simulink model "SUB_IC_Fcn_Welcome"  (R2018b)
settings: Solver=VariableStepDiscrete  StartTime=0.0  StopTime=10  RelTol=1e-3
PreLoadFcn:
  | if(exist('MBDS_ModelCallback', 'file'))
  |    MBDS_ModelCallback('PreLoad');
  | end
PostLoadFcn:
  | if(exist('MBDS_ModelCallback', 'file'))
  |    MBDS_ModelCallback('PostLoad');
  | end
InitFcn:
  | if(exist('MBDS_ModelCallback', 'file'))
  |    MBDS_ModelCallback('Init');
  | end
StartFcn:
  | if(exist('MBDS_ModelCallback', 'file'))
  |    MBDS_ModelCallback('Start');
  | end
StopFcn:
  | if(exist('MBDS_ModelCallback', 'file'))
  |    MBDS_ModelCallback('Stop');
  | end
undefined symbols (not defined in the file): nbo_False, nbo_True, sigbuilder_block
libraries: simulink x1
PreSaveFcn:
  | if(exist('MBDS_ModelCallback', 'file'))
  |    MBDS_ModelCallback('PreSave');
  | end
CloseFcn:
  | if(exist('MBDS_ModelCallback', 'file'))
  |    MBDS_ModelCallback('Close');
  | end
Description:
  | Design model of an MBDS Subsystem
settings Model: IsTargetCode=false  MBDS_Version=08.20  PauseTimes=0.1  Creator=Marcio Kopke (uid96494)  LastModifiedBy=uie79669
settings ConfigSet: Description=MBDS configuration set optimized for simulation of model designs for automotive embedded systems.
settings SolverCC: MinimalZcImpactIntegration=on
settings DataIOCC: MaxDataPoints=100  SaveFormat=StructureWithTime  SaveOutput=off  DSMLogging=off  VisualizeSimOutput=off  SaveTime=off  SignalLoggingName=LogSignals
settings OptimizationCC: UseDivisionForNetSlopeComputation=UseDivisionForReciprocalsOfIntegersOnly  UseFloatMulNetSlope=on  DefaultUnderspecifiedDataType=single  OptimizeBlockIOStorage=off  BufferReuse=off  GlobalBufferReuse=off  StrengthReduction=on  ExpressionFolding=off  ExpressionDepthLimit=2147483647  LocalBlockOutputs=off  EfficientFloat2IntCast=on  LifeSpan=inf  BufferReusableBoundary=off  OptimizeBlockOrder=speed  OptimizeDataStoreBuffers=off  BusAssignmentInplaceUpdate=off  LabelGuidedReuse=on
settings DebuggingCC: SignalInfNanChecking=error  AlgebraicLoopMsg=error  ArtificialAlgebraicLoopMsg=error  UnderspecifiedInitializationDetection=Classic  CheckExecutionContextPreStartOutputMsg=on  CheckExecutionContextRuntimeOutputMsg=on  BlockPriorityViolationMsg=error  MinStepSizeMsg=error  TimeAdjustmentMsg=warning  SolverPrmCheckMsg=error  InheritedTsInSrcMsg=none  SingleTaskRateTransMsg=error  TasksWithSamePriorityMsg=error  SigSpecEnsureSampleTimeMsg=error  CheckMatrixSingularityMsg=error  ParameterUnderflowMsg=error  ParameterTunabilityLossMsg=error  FixptConstUnderflowMsg=warning  FixptConstOverflowMsg=warning  FixptConstPrecisionLossMsg=warning  VectorMatrixConversionMsg=error  SignalLabelMismatchMsg=warning  SFcnCompatibilityMsg=error  FrameProcessingCompatibilityMsg=warning  UniqueDataStoreMsg=error  BusObjectLabelMismatch=error  RootOutportRequireBusObject=error  AllowSymbolicDim=off  ModelReferenceIOMsg=error  ModelReferenceIOMismatchMessage=error  UnknownTsInhSupMsg=error  ModelReferenceDataLoggingMessage=error  StateNameClashWarn=warning  SimStateOlderReleaseMsg=warning  StrictBusMsg=ErrorOnBusTreatedAsVector  NonBusSignalsTreatedAsBus=error  SFInvalidInputDataAccessInChartInitDiag=error  SFTransitionOutsideNaturalParentDiag=error  SFUnreachableExecutionPathDiag=error  SFUndirectedBroadcastEventsDiag=error  SFTransitionActionBeforeConditionDiag=error  SFTemporalDelaySmallerThanSampleTimeDiag=error  SFExecutionAtInitializationDiag=none
settings HardwareCC: ProdBitPerPointer=32  ProdBitPerSizeT=32  ProdBitPerPtrDiffT=32  ProdLargestAtomicInteger=Long  ProdEndianess=BigEndian  ProdWordSize=32  ProdLongLongMode=on  ProdHWDeviceType=Custom Processor  TargetHWDeviceType=32-bit Generic
settings ModelReferenceCC: PropagateSignalLabelsOutOfModel=off
settings SFSimCC: SimUseLocalCustomCode=off  SimGenImportedTypeDefs=on  CompileTimeRecursionLimit=0  EnableRuntimeRecursion=off  MATLABDynamicMemAlloc=off  DefaultCustomCodeFunctionArrayLayout=Column-major
settings RTWCC: SystemTargetFile=MBDS.tlc  GenCodeOnly=on  TemplateMakefile=MBDS.tmf  Description=MBDS Target  GenerateReport=on  RTWUseLocalCustomCode=off  IncludeHyperlinkInReport=on  LaunchReport=on  GenerateTraceReport=on  GenerateTraceReportSl=on  GenerateTraceReportSf=on  GenerateTraceReportEml=on  GenerateCodeMetricsReport=on  RTWCompilerOptimization=on
settings CodeAppCC: ForceParamTrailComments=on  IgnoreCustomStorageClasses=off  OperatorAnnotations=on  SimulinkDataObjDesc=on  SFDataObjDesc=on  MangleLength=2  CustomSymbolStrType=$N$R$M  CustomSymbolStrFcn=$R$M  CustomSymbolStrUtil=$n$C  InsertBlockDesc=on  StateflowObjectComments=on  MATLABSourceComments=on  ReqsInCode=on  UseSimReservedNames=on
settings STFCustomTargetCC: UtilityFuncGeneration=Shared location  MultiwordLength=256  DynamicStringBufferSize=2  InferredTypesCompatibility=on  ModelReferenceCompliant=off  IncludeMdlTerminateFcn=off  CombineOutputUpdateFcns=on  CombineSignalStateStructs=on  SuppressErrorStatus=on  ERTCustomFileBanners=on  SupportComplex=off  SupportContinuousTime=off  SupportNonInlinedSFcns=off  RemoveDisableFunc=on  RemoveResetFunc=on  ParenthesesLevel=Maximum  CastingMode=Standards  MATLABClassNameForMDSCustomization=Simulink.SoftwareTarget.ERTCustomization  GenerateSharedConstants=off  SystemTargetFile=MBDS.tlc
settings ERTTargetCC: UtilityFuncGeneration=Shared location  DynamicStringBufferSize=2  InferredTypesCompatibility=on  ModelReferenceCompliant=off  ParMdlRefBuildCompliant=off  CompOptLevelCompliant=off  ConcurrentExecutionCompliant=off  IncludeMdlTerminateFcn=off  CombineSignalStateStructs=on  SuppressErrorStatus=on  SupportComplex=off  RemoveDisableFunc=on  ParenthesesLevel=Maximum  CastingMode=Standards  ModelStepFunctionPrototypeControlCompliant=off  CPPClassGenCompliant=off  UseToolchainInfoCompliant=off  GenerateSharedConstants=off  ERTCustomFileTemplate=example_file_process.tlc  EnableDataOwnership=on  PreserveExpressionOrder=on  PreserveIfCondition=on  SuppressUnreachableDefaultCases=off  EnableSignedLeftShifts=off  EnableSignedRightShifts=off  IndentStyle=Allman  NewlineStyle=CR+LF
settings ConfigComp: CovScope=ReferencedModels  CovIncludeTopModel=off  CovPath=SUB_IC_Fcn_Welcome/Model/SUB_IC_Fcn_Welcome_  CovSaveName=covData  CovMetricSettings=dsw  CovFilter=MBDS_CoverageFilter  CovHTMLOptions=-sRT=1 -sVT=0 -aTS=1 -bRG=1 -bTC=1 -hTR=1 -nFC=0 -nFD=0 -scm=1 -bcm=1 -xEv=0 -xEM=1  CovHtmlReporting=on  CovSaveOutputData=off  CovDataFileName=covData  CovShowResultsExplorer=off  CovExternalEMLEnable=off  CovSFcnEnable=off

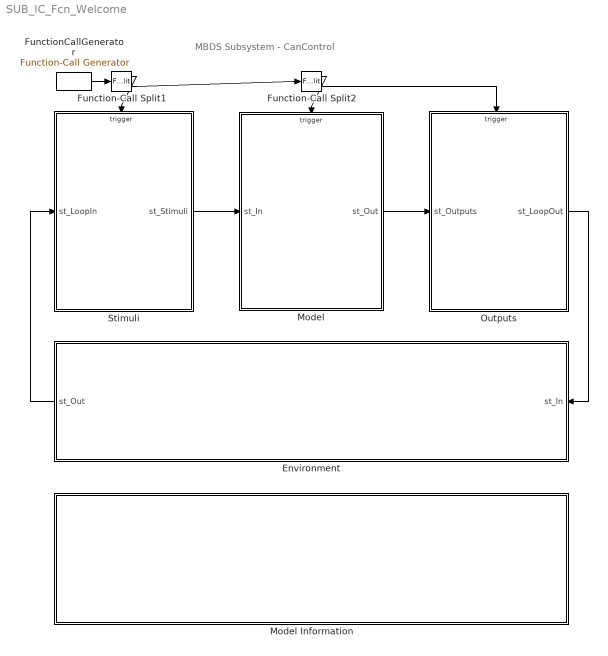
== system SUB_IC_Fcn_Welcome ==
  note: MBDS Subsystem - CanControl
  Environment : Subsystem  Description=Environment subsystem for a MBDS model.
  Function-Call Split1 : FunctionCallSplit  InitFcn=|  NumOutputPorts=2
      | try
      |    MBDS_BlockCallback('Update', gcb);
      | end
      | try
      |    MBDS_BlockCallback('Update', gcb);
      | end
  Function-Call Split2 : FunctionCallSplit  InitFcn=|  NumOutputPorts=2
      | try
      |    MBDS_BlockCallback('Update', gcb);
      | end
      | try
      |    MBDS_BlockCallback('Update', gcb);
      | end
  FunctionCallGenerator : simulink/Ports & Subsystems/Function-Call Generator  sample_time=0.01  numberOfIterations=1
      settings: AttributesFormatString=Ts = %<sample_time>
  Model : Subsystem  Description=Model subsystem for a MBDS model. Here, the input signals to the model functionality are resolved from the Stimuli bus and the output signals of the model functionality are summarized into the Results bus.
  Model Information : Subsystem  InitFcn=|  mask(ModelInformation){MBDS_LibraryBlock=on, Company=-, Department=-, Responsible=-, Status=In Work, Complete=on, Check=on, Test=on, Optimize=on, Documentation=on, FcnErrors=off, GenericToDo=off, DocumentState=Draft, GenericToDoName=Enter a user specific ToDo text, MBDS_BlockVersion=07.00}
      | if(exist('MBDS_BlockCallback', 'file'))
      |    MBDS_BlockCallback('Update', gcb);
      | end
      mask prompts: MBDS_LibraryBlock "MBDS Library Block"; Complete "Complete Implementation"; Check "Check Modelling Guidelines"; Test "Test Functionality"; Optimize "Optimize Implementation"; Documentation "Create Documentation"; FcnErrors "Remove Functional Errors"; GenericToDo "Enter a user specific ToDo text"; DocumentState "Document State:"; GenericToDoName "Generic ToDo Name:"; MBDS_BlockVersion "Block version:"
      mask help: This block displays model information and ToDo's on it's block mask. Via the block parameter mask further model information and configuration options can be accessed.
      mask init:
      | if(exist('MBDS_BlockCallback', 'file'))
      |    MBDS_BlockCallback('Copy', gcb);    
      | end
      mask Help: eval(['open([workdir(''library_dir:''),''\Blockset\help\'',get_param(gcb,''MaskType''),''.html''])'])
      mask TypeOptions Status: In Work | Done
      mask TypeOptions DocumentState: Draft | Final | Released
      mask Callback GenericToDoName:
      | MaskPrompts = get_param(gcb, 'MaskPrompts');
      | MaskPrompts{12} = get_param(gcb, 'GenericToDoName');
      | if(length(MaskPrompts{12}) > 75)
      |    MaskPrompts{12} = MaskPrompts{12}(1:75);
      |    set_param(gcb, 'GenericToDoName', MaskPrompts{12});
      | end
      | set_param(gcb, 'MaskPrompts', MaskPrompts);
      | clear MaskPrompts;
      mask DialogControl ParameterTabVar0 Prompt: Info
      mask DialogControl ParameterTabVar01 Prompt: ToDo's
      mask DialogControl ParameterTabVar012 Prompt: Options
      mask DialogControl ParameterTabVar0123 Prompt: Version
      mask Display:
      | % Get ToDo's
      | IsComplete       = strcmpi(Complete, 'on');
      | IsOptimize       = strcmpi(Optimize, 'on');
      | IsCheck          = strcmpi(Check, 'on');
      | IsDocumentation  = strcmpi(Documentation, 'on');
      | IsTest           = strcmpi(Test, 'on');
      | IsFcnErrors      = strcmpi(FcnErrors, 'on');
      | IsGenericToDo    = strcmpi(GenericToDo, 'on');
      | 
      | % Determine status
      | if(IsFcnErrors || IsTest || IsComplete || IsDocumentation || IsCheck || IsOptimize || IsGenericToDo)
      |    Status = 'In Work';
      | else
      |    Status = 'Done';
      | end
      | 
      | % Update status parameter
      | if(~strcmpi(get_param(gcb, 'Status'), Status))
      |    set_param(gcb, 'Status', Status);
      | end
      | 
      | % Determine severity
      | if(IsFcnErrors)
      |    % Severity: Critical
      |    BoxColorFile = 'Box_Red.tif';
      |    IconFile     = 'State_Red.jpg';
      | elseif (IsTest || IsComplete || IsGenericToDo)
      |    % Severity: Major
      |    BoxColorFile = 'Box_Orange.tif';
      |    IconFile     = 'State_Orange.jpg';
      | elseif (IsDocumentation || IsCheck || IsOptimize)
      |    % Severity: Minor
      |    BoxColorFile = 'Box_Grey.tif';
      |    IconFile     = 'State_Grey.jpg';
      | else
      |    % Severity: None
      |    BoxColorFile = 'Box_Green.tif';
      |    IconFile     = 'State_Green.jpg';
      | end
      | 
      | % Display Model Information
      | InfoStr1 = sprintf('%s', get_param(bdroot, 'Name'));
      | InfoStr2 = sprintf('Model Version:  %s', get_param(bdroot, 'ModelVersion'));
      | InfoStr3 = sprintf('Company:  %s', Company);
      | InfoStr4 = sprintf('Department:  %s', Department);
      | InfoStr5 = sprintf('Responsible:  %s', Responsible);
      | InfoStr6 = sprintf('Last Modified by:  %s at %s', get_param(bdroot, 'LastModifiedBy'), get_param(bdroot, 'LastModifiedDate'));
      | %Y is to do!!!!
      | text(0.5, 0.69, sprintf('%s\n%s\n%s\n%s\n%s\n%s\n%s', InfoStr1, InfoStr2, InfoStr3, InfoStr4, InfoStr5, InfoStr6), 'horizontalAlignment', 'center');
      | clear InfoStr1 InfoStr2 InfoStr3 InfoStr4 InfoStr5 InfoStr6;
      | 
      | % Display Status
      | if(exist(BoxColorFile, 'file'))
      |    image(imread(BoxColorFile,'tif'), [0,0,1,0.45]);
      | end
      | if(exist(IconFile, 'file'))
      |    image(imread(IconFile,'jpg'), [0.025,0.09,0.08,0.26]);
      |    image(imread(IconFile,'jpg'), [0.9,0.09,0.08,0.26]);
      | end
      | plot([-0.01 1.01], [0.45 0.45])
      | text(0.5, 0.38, sprintf('Status: %s', upper(Status)), 'horizontalAlignment', 'center');
      | 
      | % Display ToDo's
      | if(IsComplete)
      |    text(0.15, 0.31, '- Complete Implementation');
      | end
      | if(IsOptimize)
      |    text(0.6, 0.31, '- Optimize Implementation');
      | end
      | 
      | if(IsCheck)
      |    text(0.15, 0.23, '- Check Modeling Guidelines');
      | end
      | if(IsDocumentation)
      |    text(0.6, 0.23, '- Create Documentation');
      | end
      | 
      | if(IsTest)
      |    text(0.15, 0.14, '- Test Functionality');
      | end
      | if(IsFcnErrors)
      |    text(0.6, 0.14, '- Remove Functional Errors');
      | end
      | 
      | if(IsGenericToDo)
      |    text(0.15, 0.06, ['- ', GenericToDoName]);
      | end
  Outputs : Subsystem  Description=Result subsystem for a MBDS model. Here, output signals from the model functionality can be displayed using a scope or display. Additionally, the output signals can be postprocessed before they will passed to the feedback loop.
  Stimuli : Subsystem  Description=Stimuli subsystem for a MBDS model. Here, input signals for testing the model functionality can be defined using the signal builder or calculated applying arbitrary basic-blocks. Additionally, feedback signals can be preprocessed at this stage.
  wires:
  Model/1(st_Out) -> Outputs/1(st_Outputs)
  Stimuli/1(st_Stimuli) -> Model/1(st_In)
  Outputs/1(st_LoopOut) -> Environment/1(st_In)
  Environment/1(st_Out) -> Stimuli/1(st_LoopIn)
  FunctionCallGenerator/1 -> Function-Call Split1/1
  Function-Call Split1/2 -> Function-Call Split2/1
  Function-Call Split1/1 -> Stimuli/Trigger
  Function-Call Split2/1 -> Model/Trigger
  Function-Call Split2/2 -> Outputs/Trigger

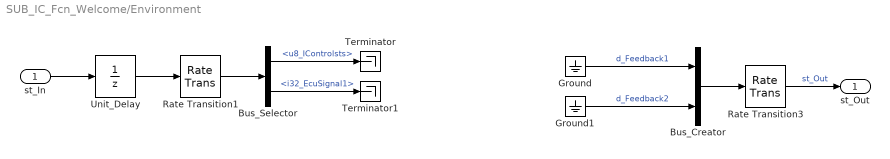
== system SUB_IC_Fcn_Welcome/Environment ==
  st_In : Inport
  Bus_Creator : BusCreator  InitFcn=|  Inputs=2
      | try
      |    MBDS_BlockCallback('Update', gcb);
      | end
      | try
      |    MBDS_BlockCallback('Update', gcb);
      | end
  Bus_Selector : BusSelector  InitFcn=|  OutputSignals=st_Outputs.u8_IControlsts,i32_EcuSignal1
      | try
      |    MBDS_BlockCallback('Update', gcb);
      | end
      | try
      |    MBDS_BlockCallback('Update', gcb);
      | end
  Ground : Ground  InitFcn=|
      | try
      |    MBDS_BlockCallback('Update', gcb);
      | end
  Ground1 : Ground  InitFcn=|
      | try
      |    MBDS_BlockCallback('Update', gcb);
      | end
  Rate Transition1 : RateTransition  InitFcn=|  OutPortSampleTimeOpt=Inherit
      | try
      |    MBDS_BlockCallback('Update', gcb);
      | end
  Rate Transition3 : RateTransition  InitFcn=|  OutPortSampleTimeOpt=Inherit
      | try
      |    MBDS_BlockCallback('Update', gcb);
      | end
  Terminator : Terminator
      settings: MoveFcn=UpdateBlockSize(gcb);
      settings: InitFcn=|
      | try
      |    MBDS_BlockCallback('Update', gcb);
      | end
  Terminator1 : Terminator
      settings: MoveFcn=UpdateBlockSize(gcb);
      settings: InitFcn=|
      | try
      |    MBDS_BlockCallback('Update', gcb);
      | end
  Unit_Delay : UnitDelay  InitFcn=|  SampleTime=-1
      | try
      |    MBDS_BlockCallback('Update', gcb);
      | end
      | try                                  
      |    MBDS_BlockCallback('Update', gcb);
      | end
      settings: AttributesFormatString=Init = %<X0>
  st_Out : Outport
  wires:
  Bus_Creator/1 -> Rate Transition3/1
  st_In/1 -> Unit_Delay/1
  Ground/1 -> Bus_Creator/1  "d_Feedback1"
  Ground1/1 -> Bus_Creator/2  "d_Feedback2"
  Unit_Delay/1 -> Rate Transition1/1
  Rate Transition3/1 -> st_Out/1  "st_Out"
  Rate Transition1/1 -> Bus_Selector/1
  Bus_Selector/1 -> Terminator/1  "<u8_IControlsts>"
  Bus_Selector/2 -> Terminator1/1  "<i32_EcuSignal1>"

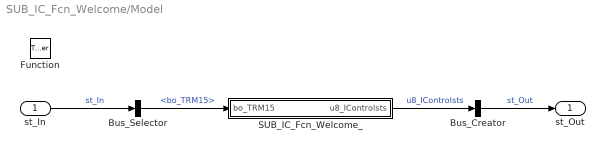
== system SUB_IC_Fcn_Welcome/Model ==
  st_In : Inport
      settings: LatchInputForFeedbackSignals=on
  Function : TriggerPort  InitFcn=|  TriggerType=function-call  VariantControl=(inherit)
      | try
      |    MBDS_BlockCallback('Update', gcb);
      | end
  Bus_Creator : BusCreator  InitFcn=|  Inputs=1
      | try
      |    MBDS_BlockCallback('Update', gcb);
      | end
      | try
      |    MBDS_BlockCallback('Update', gcb);
      | end
  Bus_Selector : BusSelector  InitFcn=|  OutputSignals=bo_TRM15
      | try
      |    MBDS_BlockCallback('Update', gcb);
      | end
      | try
      |    MBDS_BlockCallback('Update', gcb);
      | end
  SUB_IC_Fcn_Welcome_ : Subsystem  Tag=Functionality  Description=CAN Control
      settings: AttributesFormatString=Functionality
  st_Out : Outport
  wires:
  st_In/1 -> Bus_Selector/1  "st_In"
  Bus_Creator/1 -> st_Out/1  "st_Out"
  Bus_Selector/1 -> SUB_IC_Fcn_Welcome_/1(bo_TRM15)  "<bo_TRM15>"
  SUB_IC_Fcn_Welcome_/1(u8_IControlsts) -> Bus_Creator/1  "u8_IControlsts"

== system SUB_IC_Fcn_Welcome/Model Information ==
  note: Double Click the Model Information block to open the block parameter mask

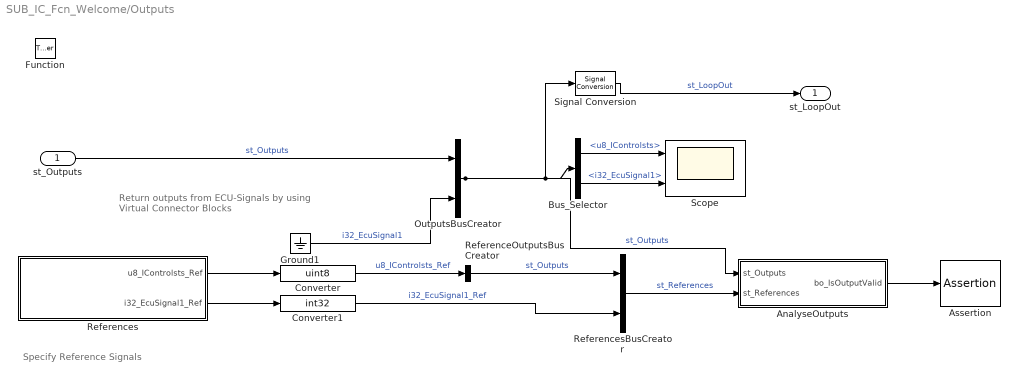
== system SUB_IC_Fcn_Welcome/Outputs ==
  note: Specify Reference Signals
  note: Return outputs from ECU-Signals
      | by using Virtual Connector Blocks
  st_Outputs : Inport
      settings: LatchInputForFeedbackSignals=on
  Function : TriggerPort  InitFcn=|  TriggerType=function-call  VariantControl=(inherit)
      | try
      |    MBDS_BlockCallback('Update', gcb);
      | end
  AnalyseOutputs : Subsystem
  Assertion : Assertion  Enabled=off
  Bus_Selector : BusSelector  InitFcn=|  OutputSignals=st_Outputs.u8_IControlsts,i32_EcuSignal1
      | try
      |    MBDS_BlockCallback('Update', gcb);
      | end
      | try
      |    MBDS_BlockCallback('Update', gcb);
      | end
  Converter : DataTypeConversion  InitFcn=|  OutDataTypeStr=uint8  SaturateOnIntegerOverflow=on
      | try
      |    MBDS_BlockCallback('Update', gcb);
      | end
      settings: AttributesFormatString=Saturate: %<SaturateOnIntegerOverflow>
  Converter1 : DataTypeConversion  InitFcn=|  OutDataTypeStr=int32  SaturateOnIntegerOverflow=on
      | try
      |    MBDS_BlockCallback('Update', gcb);
      | end
      settings: AttributesFormatString=Saturate: %<SaturateOnIntegerOverflow>
  Ground1 : Ground  InitFcn=|
      | try
      |    MBDS_BlockCallback('Update', gcb);
      | end
      | try
      |    MBDS_BlockCallback('Update', gcb);
      | end
  OutputsBusCreator : BusCreator  InitFcn=|  Inputs=2
      | try
      |    MBDS_BlockCallback('Update', gcb);
      | end
      | try
      |    MBDS_BlockCallback('Update', gcb);
      | end
  ReferenceOutputsBusCreator : BusCreator  InitFcn=|  Inputs=1
      | try
      |    MBDS_BlockCallback('Update', gcb);
      | end
      | try
      |    MBDS_BlockCallback('Update', gcb);
      | end
  References : Subsystem  Tag=STV Subsys  LoadFcn=sigbuilder_block('load');  StartFcn=sigbuilder_block('start');  StopFcn=sigbuilder_block('stop');  ClipboardFcn=sigbuilder_block('clipboard');  mask(Sigbuilder block){tuvar=[0:10]}
      mask init:
      | if ~strcmp(get_param(bdroot(gcb),'SimulationStatus'),'stopped'),tuvar = sigbuilder_block('maskInit'); end
      settings: CopyFcn=sigbuilder_block('copy');  DeleteFcn=sigbuilder_block('delete');  ModelCloseFcn=sigbuilder_block('modelClose');  PreSaveFcn=sigbuilder_block('preSave');  PauseFcn=sigbuilder_block('pause');  ContinueFcn=sigbuilder_block('continue');  NameChangeFcn=sigbuilder_block('namechange');  OpenFcn=sigbuilder_block('open',[50 50 520 400 ]);  CloseFcn=sigbuilder_block('close');
      mask Display: plot(0, 0, 100, 100,[2, 2, 32, 32, 2], [68, 8, 8, 68, 68],[32, 2], [38, 38], [32, 19, 2],[53, 60, 44], [32, 17, 17, 2],[16, 16, 31, 31]);txt = getActiveGroup(gcbh);text(2, 100, txt,'verticalAlignment', 'top');
  ReferencesBusCreator : BusCreator  InitFcn=|  Inputs=2
      | try
      |    MBDS_BlockCallback('Update', gcb);
      | end
      | try
      |    MBDS_BlockCallback('Update', gcb);
      | end
  Scope : Scope  NumInputPorts=2
  Signal Conversion : SignalConversion  InitFcn=|  OverrideOpt=off
      | try
      |    MBDS_BlockCallback('Update', gcb);
      | end
  st_LoopOut : Outport
  wires:
  AnalyseOutputs/1(bo_IsOutputValid) -> Assertion/1
  ReferencesBusCreator/1 -> AnalyseOutputs/2(st_References)  "st_References"
  st_Outputs/1 -> OutputsBusCreator/1  "st_Outputs"
  Ground1/1 -> OutputsBusCreator/2  "i32_EcuSignal1"
  OutputsBusCreator/1 -> Signal Conversion/1, Bus_Selector/1, AnalyseOutputs/1(st_Outputs)  "st_Outputs"
  Signal Conversion/1 -> st_LoopOut/1  "st_LoopOut"
  Bus_Selector/1 -> Scope/1  "<u8_IControlsts>"
  Bus_Selector/2 -> Scope/2  "<i32_EcuSignal1>"
  ReferenceOutputsBusCreator/1 -> ReferencesBusCreator/1  "st_Outputs"
  Converter/1 -> ReferenceOutputsBusCreator/1  "u8_IControlsts_Ref"
  References/1(u8_IControlsts_Ref) -> Converter/1
  References/2(i32_EcuSignal1_Ref) -> Converter1/1
  Converter1/1 -> ReferencesBusCreator/2  "i32_EcuSignal1_Ref"

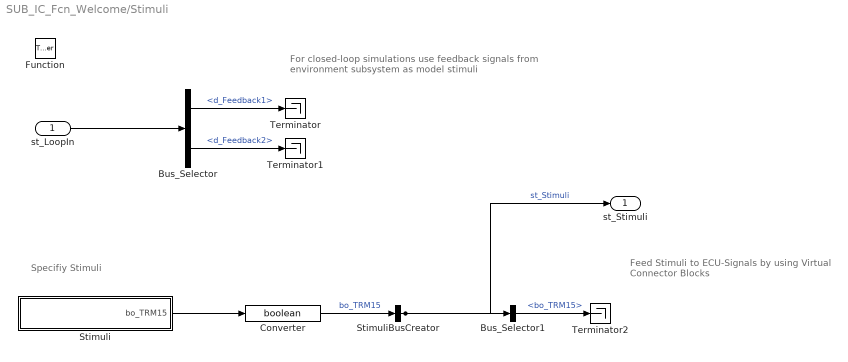
== system SUB_IC_Fcn_Welcome/Stimuli ==
  note: Specifiy Stimuli
  note: For closed-loop simulations use feedback signals
      | from environment subsystem as model stimuli
  note: Feed Stimuli to ECU-Signals
      | by using Virtual Connector Blocks
  st_LoopIn : Inport
      settings: LatchInputForFeedbackSignals=on
  Function : TriggerPort  InitFcn=|  TriggerType=function-call  VariantControl=(inherit)
      | try
      |    MBDS_BlockCallback('Update', gcb);
      | end
  Bus_Selector : BusSelector  InitFcn=|  OutputSignals=d_Feedback1,d_Feedback2
      | try
      |    MBDS_BlockCallback('Update', gcb);
      | end
      | try
      |    MBDS_BlockCallback('Update', gcb);
      | end
  Bus_Selector1 : BusSelector  InitFcn=|  OutputSignals=bo_TRM15
      | try
      |    MBDS_BlockCallback('Update', gcb);
      | end
      | try
      |    MBDS_BlockCallback('Update', gcb);
      | end
  Converter : DataTypeConversion  InitFcn=|  OutDataTypeStr=boolean  SaturateOnIntegerOverflow=on
      | try
      |    MBDS_BlockCallback('Update', gcb);
      | end
      settings: AttributesFormatString=Saturate: %<SaturateOnIntegerOverflow>
  Stimuli : Subsystem  Tag=STV Subsys  LoadFcn=sigbuilder_block('load');  StartFcn=sigbuilder_block('start');  StopFcn=sigbuilder_block('stop');  ClipboardFcn=sigbuilder_block('clipboard');  mask(Sigbuilder block){tuvar=[0:10]}
      mask init:
      | if ~strcmp(get_param(bdroot(gcb),'SimulationStatus'),'stopped'),tuvar = sigbuilder_block('maskInit'); end
      settings: CopyFcn=sigbuilder_block('copy');  DeleteFcn=sigbuilder_block('delete');  ModelCloseFcn=sigbuilder_block('modelClose');  PreSaveFcn=sigbuilder_block('preSave');  PauseFcn=sigbuilder_block('pause');  ContinueFcn=sigbuilder_block('continue');  NameChangeFcn=sigbuilder_block('namechange');  OpenFcn=sigbuilder_block('open',[50 50 520 400 ]);  CloseFcn=sigbuilder_block('close');
      mask Display: plot(0, 0, 100, 100,[2, 2, 32, 32, 2], [68, 8, 8, 68, 68],[32, 2], [38, 38], [32, 19, 2],[53, 60, 44], [32, 17, 17, 2],[16, 16, 31, 31]);txt = getActiveGroup(gcbh);text(2, 100, txt,'verticalAlignment', 'top');
  StimuliBusCreator : BusCreator  InitFcn=|  Inputs=1
      | try
      |    MBDS_BlockCallback('Update', gcb);
      | end
      | try
      |    MBDS_BlockCallback('Update', gcb);
      | end
  Terminator : Terminator
      settings: InitFcn=|
      | try
      |    MBDS_BlockCallback('Update', gcb);
      | end
      | try
      |    MBDS_BlockCallback('Update', gcb);
      | end
  Terminator1 : Terminator
      settings: InitFcn=|
      | try
      |    MBDS_BlockCallback('Update', gcb);
      | end
      | try
      |    MBDS_BlockCallback('Update', gcb);
      | end
  Terminator2 : Terminator
      settings: MoveFcn=UpdateBlockSize(gcb);
      settings: InitFcn=|
      | try
      |    MBDS_BlockCallback('Update', gcb);
      | end
  st_Stimuli : Outport
  wires:
  Bus_Selector/1 -> Terminator/1  "<d_Feedback1>"
  Bus_Selector/2 -> Terminator1/1  "<d_Feedback2>"
  st_LoopIn/1 -> Bus_Selector/1
  Bus_Selector1/1 -> Terminator2/1  "<bo_TRM15>"
  StimuliBusCreator/1 -> Bus_Selector1/1, st_Stimuli/1  "st_Stimuli"
  Converter/1 -> StimuliBusCreator/1  "bo_TRM15"
  Stimuli/1(bo_TRM15) -> Converter/1

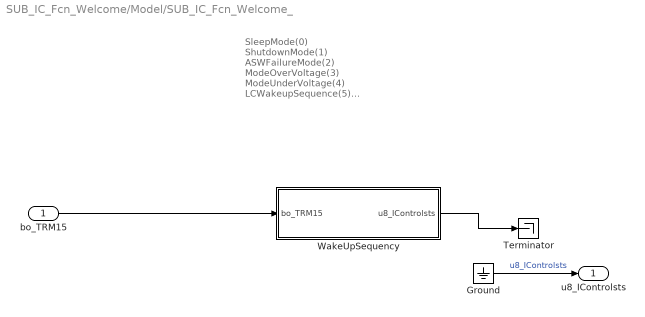
== system SUB_IC_Fcn_Welcome/Model/SUB_IC_Fcn_Welcome_ ==
  note: SleepMode(0)
      | ShutdownMode(1)
      | ASWFailureMode(2)
      | ModeOverVoltage(3)
      | ModeUnderVoltage(4)
      | LCWakeupSequence(5)
      | TimeoutFailureMode(6)
      |  ActiveMode(7)
      |  SYFlashingMode(8)
  bo_TRM15 : Inport  Description=Receive the signal status KL15, ON/OFF  OutDataTypeStr=boolean
  Ground : Ground  InitFcn=|
      | try
      |    MBDS_BlockCallback('Update', gcb);
      | end
      settings: MoveFcn=UpdateBlockSize(gcb);
  Terminator : Terminator
      settings: MoveFcn=UpdateBlockSize(gcb);
      settings: InitFcn=|
      | try
      |    MBDS_BlockCallback('Update', gcb);
      | end
  WakeUpSequency : Stateflow chart  TreatAsAtomicUnit=on
      settings: CopyFcn=|
      | if(exist('MBDS_BlockCallback', 'file'))
      |    MBDS_BlockCallback('Copy', gcb);
      | end
  u8_IControlsts : Outport  Description=Send to Cluster the signal Status  OutDataTypeStr=uint8
  wires:
  bo_TRM15/1 -> WakeUpSequency/1(bo_TRM15)
  WakeUpSequency/1(u8_IControlsts) -> Terminator/1
  Ground/1 -> u8_IControlsts/1  "u8_IControlsts"

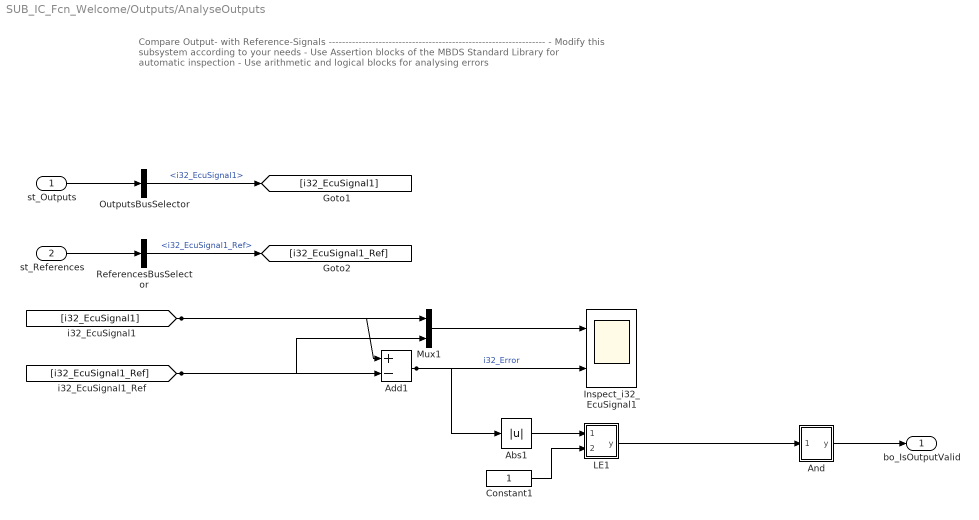
== system SUB_IC_Fcn_Welcome/Outputs/AnalyseOutputs ==
  note: Compare Output- with Reference-Signals
      | -----------------------------------------------------------------
      | - Modify this subsystem according to your needs
      | -  Use Assertion blocks of the MBDS Standard Library for automatic inspection
      | - Use arithmetic and logical blocks for analysing errors
  st_Outputs : Inport  InitFcn=|
      | try
      |    MBDS_BlockCallback('Update', gcb);
      | end
  st_References : Inport  InitFcn=|  Port=2
      | try
      |    MBDS_BlockCallback('Update', gcb);
      | end
  Abs1 : Abs  InitFcn=|  OutDataTypeStr=Inherit: Inherit via back propagation
      | if(exist('MBDS_BlockCallback', 'file'))
      |    MBDS_BlockCallback('Update', gcb);  
      | end
      settings: AttributesFormatString=Saturate: %<SaturateOnIntegerOverflow>
  Add1 : Sum  InitFcn=|  Inputs=+-  OutDataTypeStr=int32  SaturateOnIntegerOverflow=on  InputSameDT=on
      | if(exist('MBDS_BlockCallback', 'file'))
      |    MBDS_BlockCallback('Update', gcb);  
      | end
      settings: AttributesFormatString=Saturate: %<SaturateOnIntegerOverflow>
  And : Subsystem  InitFcn=|  mask(AND){MBDS_LibraryBlock=on, BitwiseMode=off, Inputs=1, UseBitMask=off, BitMask='A7', OutDataTypeStr=Inherit: Inherit via back propagation, MBDS_BlockVersion=08.20.05}
      | if(exist('MBDS_BlockCallback', 'file'))
      |    MBDS_BlockCallback('Update', gcb);
      | end
      mask prompts: MBDS_LibraryBlock "MBDS library block"; BitwiseMode "Use 'bitwise' mode"; Inputs "Number of input ports:"; UseBitMask "Use bit mask"; BitMask "Bit mask:"; OutDataTypeStr "Output data type:"; MBDS_BlockVersion "Version:"
      mask help: Logical or bitwise AND operator. For multiple inputs, operators are applied across the inputs. For a single input, operators are applied across the input vector. In bitwise mode a bit mask can be applied onto single input signals.
      mask init:
      | if(exist('MBDS_BlockCallback', 'file'))
      |    MBDS_BlockCallback('Init', gcb);
      | else
      |    % Disable all mask parameters
      |    MaskEnables = get_param(gcb, 'MaskEnables');
      |    for k = [1:length(MaskEnables)]
      |       MaskEnables{k} = 'off';
      |    end
      |    if(~isequal(MaskEnables, get_param(gcb, 'MaskEnables')))
      |       set_param(gcb, 'MaskEnables', MaskEnables);
      |    end
      | end
      mask Help: eval(['open([workdir(''library_dir:''),''\Blockset\help\'',get_param(gcb,''MaskType''),''.html''])'])
      mask Callback BitwiseMode:
      | if(exist('MBDS_BlockCallback', 'file'))
      |    MBDS_BlockCallback('BitwiseMode', gcb);
      | end
      mask Callback Inputs:
      | if(exist('MBDS_BlockCallback', 'file'))
      |    MBDS_BlockCallback('Inputs', gcb);
      | end
      mask Callback UseBitMask:
      | if(exist('MBDS_BlockCallback', 'file'))
      |    MBDS_BlockCallback('UseBitMask', gcb);
      | end
      mask Callback BitMask:
      | if(exist('MBDS_BlockCallback', 'file'))
      |    MBDS_BlockCallback('BitMask', gcb);
      | end
      mask TypeOptions OutDataTypeStr: Inherit: Inherit via back propagation | int8 | uint8 | int16 | uint16 | int32 | uint32 | boolean
      mask Callback OutDataTypeStr:
      | % Adopt Value
      | if(exist('MBDS_BlockCallback', 'file'))
      |    MBDS_BlockCallback('OutDataTypeStr', gcb);
      | end
      mask DialogControl ParameterTabVar0 Prompt: Main
      mask DialogControl ParameterTabVar01 Prompt: Signal Attributes
      mask DialogControl ParameterTabVar012 Prompt: Version
      mask Display:
      | % Show icon or block text
      | if(UseBitMask)
      |    if(isnumeric(BitMask))
      |       BitMaskString = ['0x',dec2hex(floor(BitMask))];
      |    elseif(ischar(BitMask))
      |       BitMaskString = ['0x',upper(BitMask)];
      |    else
      |       BitMaskString = '???';
      |    end
      |    disp(sprintf(['AND\n', BitMaskString]))
      | else
      |    disp('AND')
      | end
  Constant1 : Constant  InitFcn=|  OutDataTypeStr=Inherit: Inherit via back propagation
      | if(exist('MBDS_BlockCallback', 'file'))
      |    MBDS_BlockCallback('Update', gcb);  
      | end
  Inspect_i32_EcuSignal1 : Scope  NumInputPorts=2
  LE1 : Subsystem  InitFcn=|  mask(LE){MBDS_LibraryBlock=on, InputSameDT=on, MBDS_BlockVersion=05.20}
      | if(exist('MBDS_BlockCallback', 'file'))
      |    MBDS_BlockCallback('Update', gcb);
      | end
      mask prompts: MBDS_LibraryBlock "MBDS library block"; InputSameDT "Require all inputs to have the same data type"; MBDS_BlockVersion "Block version:"
      mask help: The block compares if the first input signal is lower than or equal to the second input signal.
      mask init: same as SUB_IC_Fcn_Welcome/Outputs/AnalyseOutputs/And
      mask Help: eval(['open([workdir(''library_dir:''),''\Blockset\help\'',get_param(gcb,''MaskType''),''.html''])'])
      mask Callback InputSameDT:
      | % Adopt value
      | if(exist('MBDS_BlockCallback', 'file'))
      |    MBDS_BlockCallback('InputSameDT', gcb);
      | end
      mask DialogControl ParameterTabVar0 Prompt: Signal Attributes
      mask DialogControl ParameterTabVar01 Prompt: Version
      mask Display:
      | % Show icon or block text
      | if(exist('MBDS_BlockCallback', 'file'))
      |    image(imread('LE.tif','tif'),[0.33,0.33,0.37,0.37])
      |    disp('')
      | else
      |    disp(sprintf('<='));
      | end
  Mux1 : Mux  InitFcn=|  Inputs=2
      | try
      |    MBDS_BlockCallback('Update', gcb);
      | end
  OutputsBusSelector : BusSelector  InitFcn=|  OutputSignals=i32_EcuSignal1
      | try
      |    MBDS_BlockCallback('Update', gcb);
      | end
  ReferencesBusSelector : BusSelector  InitFcn=|  OutputSignals=i32_EcuSignal1_Ref
      | try
      |    MBDS_BlockCallback('Update', gcb);
      | end
  bo_IsOutputValid : Outport  InitFcn=|  PortDimensions=1
      | try
      |    MBDS_BlockCallback('Update', gcb);
      | end
  wires:
  st_Outputs/1 -> OutputsBusSelector/1
  OutputsBusSelector/1 -> [i32_EcuSignal1]  "<i32_EcuSignal1>"
  st_References/1 -> ReferencesBusSelector/1
  ReferencesBusSelector/1 -> [i32_EcuSignal1_Ref]  "<i32_EcuSignal1_Ref>"
  [i32_EcuSignal1_Ref] -> Add1/2, Mux1/2
  [i32_EcuSignal1] -> Add1/1, Mux1/1
  Mux1/1 -> Inspect_i32_EcuSignal1/1
  Add1/1 -> Abs1/1, Inspect_i32_EcuSignal1/2  "i32_Error"
  Abs1/1 -> LE1/1(u1)
  Constant1/1 -> LE1/2(u2)
  And/1(y) -> bo_IsOutputValid/1
  LE1/1(y) -> And/1(u1)

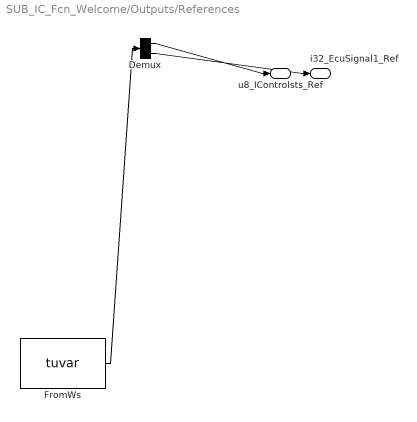
== system SUB_IC_Fcn_Welcome/Outputs/References ==
  Demux : Demux  Tag=STV Demux  Outputs=2
  FromWs : FromWorkspace  Tag=STV FromWs  VariableName=tuvar
      SigBuilderData=|
      | dataSet.timeRange = [0 10]
      | dataSet.name = 'TC1'
      | sbobj.Name = 'Signal Builder'
      | sbobj.Groups.Name = 'TC1'
      | sbobj.Groups.Signals(1).Name = 'u8_IControlsts_Ref'
      | sbobj.Groups.Signals(1).XData = [0 1 2 3 4 5 6 7 8 9 10]
      | sbobj.Groups.Signals(1).YData = [1 1 1 1 1 1 1 1 1 1 1]
      | sbobj.Groups.Signals(2).Name = 'i32_EcuSignal1_Ref'
      | sbobj.Groups.Signals(2).XData = [0 1 2 3 4 5 6 7 8 9 10]
      | sbobj.Groups.Signals(2).YData = [1 1 1 1 1 1 1 1 1 1 1]
  u8_IControlsts_Ref : Outport  Tag=STV Outport
  i32_EcuSignal1_Ref : Outport  Tag=STV Outport  Port=2
  wires:
  FromWs/1 -> Demux/1
  Demux/1 -> u8_IControlsts_Ref/1
  Demux/2 -> i32_EcuSignal1_Ref/1

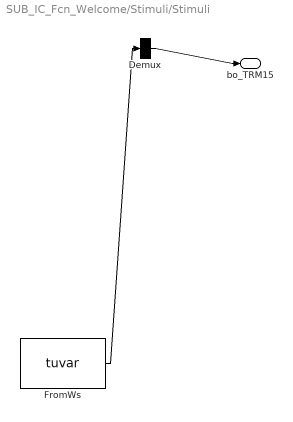
== system SUB_IC_Fcn_Welcome/Stimuli/Stimuli ==
  Demux : Demux  Tag=STV Demux  Outputs=1
  FromWs : FromWorkspace  Tag=STV FromWs  VariableName=tuvar
      SigBuilderData=|
      | dataSet.timeRange = [0 10]
      | dataSet.name = 'TC1'
      | sbobj.Name = 'Signal Builder'
      | sbobj.Groups.Name = 'TC1'
      | sbobj.Groups.Signals.Name = 'bo_TRM15'
      | sbobj.Groups.Signals.XData = [0 1 2 3 4 4 5 6 6 7 8 9 10]
      | sbobj.Groups.Signals.YData = [0 0 0 0 0 1 1 1 0 0 0 0 0]
  bo_TRM15 : Outport  Tag=STV Outport
  wires:
  FromWs/1 -> Demux/1
  Demux/1 -> bo_TRM15/1

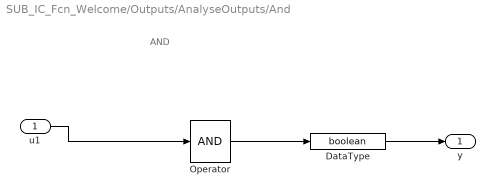
== system SUB_IC_Fcn_Welcome/Outputs/AnalyseOutputs/And ==
  note: AND
  u1 : Inport  OutDataTypeStr=boolean
  DataType : DataTypeConversion  OutDataTypeStr=boolean
  Operator : Logic  Inputs=1  AllPortsSameDT=off  OutDataTypeStr=boolean
  y : Outport
  wires:
  Operator/1 -> DataType/1
  u1/1 -> Operator/1
  DataType/1 -> y/1

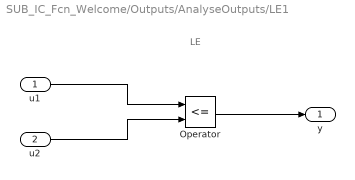
== system SUB_IC_Fcn_Welcome/Outputs/AnalyseOutputs/LE1 ==
  note: LE
  u1 : Inport
  u2 : Inport  Port=2
  Operator : RelationalOperator  Operator=<=  OutDataTypeStr=boolean  RndMeth=Nearest  InputSameDT=on
  y : Outport
  wires:
  Operator/1 -> y/1
  u2/1 -> Operator/2
  u1/1 -> Operator/1

== stateflow chart SUB_IC_Fcn_Welcome/Model/SUB_IC_Fcn_Welcome_/WakeUpSequency ==
  note: SleepMode(0)
      |       ShutdownMode(1)
      |       ASWFailureMode(2)
      |       ModeOverVoltage(3)
      |       ModeUnderVoltage(4)
      |       LCWakeupSequence(5)
      |       TimeoutFailureMode(6)
      |       ActiveMode(7)
      |       SYFlashingMode(8)
  state SleepMode
    en:
    u8_Timer = uint8(0);
    u8_IControlsts = uint8(0);
    du:
    u8_Timer ++;
  state Wakeup
    en:
    u8_IControlsts = uint8(5);
    du:
    u8_Timer ++;
  state ActiveMode
    en:
    u8_IControlsts = uint8(7);
    u8_Timer = uint8(0);
  (default) -> SleepMode
  ActiveMode -> SleepMode : [bo_TRM15 == nbo_False]
  SleepMode -> Wakeup : //Counter timer
      | [(u8_Timer >= uint8(50)) && ...
      |  (bo_TRM15 == nbo_True)]
  Wakeup -> ActiveMode : //Counter timer
      | [u8_Timer >= uint8(100)]
  data: u8_IControlsts output uint8; bo_TRM15 input boolean; nbo_True parameter boolean; nbo_False parameter boolean; u8_Timer local uint8
